simulink model "engine"  (R2019b)
settings: Solver=VariableStepAuto  StartTime=0.0  StopTime=9  MaxStep=1e-2  RelTol=1e-3
libraries: cstblocks x18, simulink x1
(part 1 of 2)
settings Model: PauseTimes=50  PacingRate=3  OrderedModelArguments=off  Creator=lenovo  LastModifiedBy=lenovo

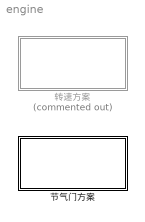
== system engine ==
  节气门方案 : Subsystem
  转速方案 : Subsystem  Commented=on

== system engine/节气门方案 ==
  note: 各个功率条件下，需要寻找功率随节气门开度变化斜率一致的转速
      | 详见转速-功率标定模块注释
  Gain : Gain  Gain=-1
  Gain1 : Gain  Gain=1e3
  Manual Switch1 : ManualSwitch
  Mux1 : Mux  Inputs=2
  Rate Limiter : RateLimiter  RisingSlewLimit=500  FallingSlewLimit=-500  SampleTimeMode=inherited
  Rate Limiter1 : RateLimiter  RisingSlewLimit=2000  FallingSlewLimit=-2000  SampleTimeMode=inherited
  Scope : Scope  NumInputPorts=4
  Sine Wave : Sin  Amplitude=10  Bias=20  Frequency=2*pi*0.01  SampleTime=0
  功率反馈补偿 : Subsystem
  功率设定 : Step  Time=3  Before=15  After=20  SampleTime=0
  功率闭环 : Subsystem  mask{Acc_p=1, Acc_n=1, Kp=3, Ki=0, Kd=0.01, D_Fc=2}
      mask prompts: Acc_p "最大正向加速度"; Acc_n "最大负向加速度"; Kp "PID-P"; Ki "PID-I"; Kd "PID-D"; D_Fc "PID-微分截止频率"
  发电机 : Subsystem
  总行程时间 : Constant  Value=3
  汽油机 : Subsystem
  电动油门 : Subsystem  mask{Deadband=1}
      mask prompts: Deadband "机械间隙（油门百分比）"
  转速-功率曲线 : Lookup_n-D  NumberOfTableDimensions=1  BreakpointsForDimension1=[0,4200,5600,6600,12500,14500,20000,26200,30500,33000]  BreakpointsForDimension2=[1:3]  Table=[800,800,860.1641,922.0328,1396.2121,1589.3308,2190.3409,2826.7045,3500,4000]  InternalRulePriority=Speed  RndMeth=Simplest  InputSameDT=on
  转速-功率标定 : Subsystem  Commented=on
  转速闭环 : Subsystem  mask{Trq_p=0, Trq_n=500, Kp=0.5, Ki=0.3, Kd=0.003, D_Fc=10}
      mask prompts: Trq_p "最大驱动扭矩"; Trq_n "最大发电扭矩"; Kp "PID-P"; Ki "PID-I"; Kd "PID-D"; D_Fc "PID-微分截止频率"
  wires:
  发电机/1(实际发电功率) -> Mux1/1, 转速-功率标定/1(发电功率)
  发电机/3(转速反馈) -> 功率反馈补偿/2(转速反馈), 转速闭环/1(转速反馈)
  发电机/2(电机实际扭矩) -> Gain/1
  汽油机/1(Speed) -> Scope/2, 发电机/1(转速)  "rpm"
  Gain/1 -> Scope/3, 汽油机/2(Load)  "负载"
  发电机/4(功率反馈) -> 功率反馈补偿/1(功率反馈)
  功率反馈补偿/1(补偿输出) -> 功率闭环/2(功率反馈)
  Gain1/1 -> Rate Limiter1/1
  Mux1/1 -> Scope/4  "功率"
  总行程时间/1 -> 电动油门/1(总行程时间)
  Rate Limiter1/1 -> 转速-功率曲线/1, 功率闭环/1(功率设定), Mux1/2
  功率闭环/1(节气门变化率输出) -> 电动油门/2(转速设定)  "油门信号"
  电动油门/1(节气门开度) -> Scope/1, 汽油机/1(Throttle)  "油门"
  转速闭环/1(扭矩输出) -> 发电机/2(扭矩设定)
  转速-功率曲线/1 -> Rate Limiter/1
  Rate Limiter/1 -> 转速闭环/2(转速设定)
  Sine Wave/1 -> Manual Switch1/1
  功率设定/1 -> Manual Switch1/2
  Manual Switch1/1 -> Gain1/1

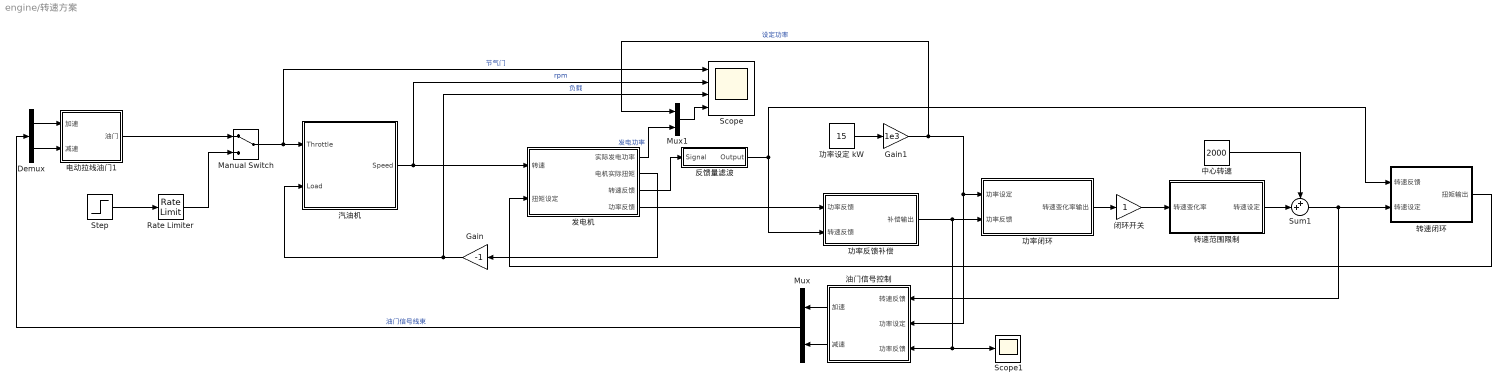
== system engine/转速方案 ==
  Demux : Demux  Outputs=2
  Gain : Gain  Gain=-1
  Gain1 : Gain  Gain=1e3
  Manual Switch : ManualSwitch
  Mux : Mux  Inputs=2
  Mux1 : Mux  Inputs=2
  Rate Limiter : RateLimiter  RisingSlewLimit=0.002  FallingSlewLimit=-0.002  SampleTimeMode=inherited
  Scope : Scope  NumInputPorts=4
  Scope1 : Scope
  Step : Step  Time=5  Before=0.2  After=0.4  SampleTime=0
  Sum1 : Sum  Inputs=++|
  中心转速 : Constant  Value=2000
  功率反馈补偿 : Subsystem
  功率设定 kW : Constant  Value=15
  功率闭环 : Subsystem  mask{Acc_p=500, Acc_n=500, Kp=0.4, Ki=0.2, Kd=0, D_Fc=20}
      mask prompts: Acc_p "最大正向加速度"; Acc_n "最大负向加速度"; Kp "PID-P"; Ki "PID-I"; Kd "PID-D"; D_Fc "PID-微分截止频率"
  反馈量滤波 : Subsystem  mask{Frq=20, Order=1}
      mask prompts: Frq "Frq_Set"; Order "Order_Set"
  发电机 : Subsystem
  汽油机 : Subsystem
  油门信号控制 : Subsystem
  电动拉线油门1 : Subsystem
  转速范围限制 : Subsystem  mask{Spe_Add=1000, Spe_Sub=1000}
      mask prompts: Spe_Add "最大转速增加量"; Spe_Sub "最大转速减少量"
  转速闭环 : Subsystem  mask{Trq_p=-10, Trq_n=500, Kp=0.8, Ki=0.7, Kd=0.005, D_Fc=20}
      mask prompts: Trq_p "最大驱动扭矩"; Trq_n "最大发电扭矩"; Kp "PID-P"; Ki "PID-I"; Kd "PID-D"; D_Fc "PID-微分截止频率"
  闭环开关 : Gain
  wires:
  Sum1/1 -> 油门信号控制/1(转速反馈), 转速闭环/2(转速设定)
  Step/1 -> Rate Limiter/1
  Mux1/1 -> Scope/4
  Gain1/1 -> Mux1/1, 功率闭环/1(功率设定), 油门信号控制/2(功率设定)  "设定功率"
  Rate Limiter/1 -> Manual Switch/2
  Manual Switch/1 -> Scope/1, 汽油机/1(Throttle)  "节气门"
  功率反馈补偿/1(补偿输出) -> 功率闭环/2(功率反馈), Scope1/1, 油门信号控制/3(功率反馈)
  油门信号控制/2(减速) -> Mux/2
  Mux/1 -> Demux/1  "油门信号线束"
  油门信号控制/1(加速) -> Mux/1
  发电机/4(功率反馈) -> 功率反馈补偿/1(功率反馈)
  闭环开关/1 -> 转速范围限制/1(转速变化率)
  Gain/1 -> 汽油机/2(Load), Scope/3  "负载"
  汽油机/1(Speed) -> Scope/2, 发电机/1(转速)  "rpm"
  发电机/2(电机实际扭矩) -> Gain/1
  发电机/3(转速反馈) -> 反馈量滤波/1(Signal)
  Demux/2 -> 电动拉线油门1/2(减速)
  转速闭环/1(扭矩输出) -> 发电机/2(扭矩设定)
  Demux/1 -> 电动拉线油门1/1(加速)
  反馈量滤波/1(Output) -> 转速闭环/1(转速反馈), 功率反馈补偿/2(转速反馈)
  功率闭环/1(转速变化率输出) -> 闭环开关/1
  中心转速/1 -> Sum1/1
  转速范围限制/1(转速设定) -> Sum1/2
  功率设定 kW/1 -> Gain1/1
  电动拉线油门1/1(油门) -> Manual Switch/1
  发电机/1(实际发电功率) -> Mux1/2  "发电功率"

== system engine/节气门方案/功率反馈补偿 ==
  note: 通过计算，将控制发动机加减速消耗的功率从功率反馈量中剔除
  note: 反馈系数：
      | 通过调整反馈系数，完全抵消转速变化时的动能变化对功率反馈的影响
      | 节气门不变，转速提高时用于反馈的功率应单调增大
      | 由于加减速时发动机工况有差异，此处反馈系数仅根据发动机转动惯量计算反馈补偿量不够准确，
      | 需要调参使得反馈效果最好。
  功率反馈 : Inport
  转速反馈 : Inport  Port=2
  Derivative : Derivative  CoefficientInTFapproximation=0.1
  Gain1 : Gain  Gain=pi/30
  Mux : Mux  Inputs=2
  Scope2 : Scope  NumInputPorts=3
  Sum : Sum  Inputs=++|
  功率反馈滤波 : Subsystem  mask{Frq=20, Order=1}
      mask prompts: Frq "Frq_Set"; Order "Order_Set"
  功率反馈补偿后滤波 : Subsystem  mask{Frq=10, Order=5}
      mask prompts: Frq "Frq_Set"; Order "Order_Set"
  反馈系数 : Gain  Gain=0.8
  转动动能 : Fcn  Expr=0.5*u(2)*u(1)*u(1)
  转动惯量 : Constant  Value=0.25
  补偿输出 : Outport
  wires:
  功率反馈/1 -> 功率反馈滤波/1(Signal)
  转动惯量/1 -> Mux/2
  Derivative/1 -> 反馈系数/1
  转速反馈/1 -> Gain1/1
  功率反馈滤波/1(Output) -> Scope2/1, Sum/1
  Mux/1 -> 转动动能/1
  转动动能/1 -> Derivative/1
  反馈系数/1 -> Sum/2, Scope2/2
  Sum/1 -> 功率反馈补偿后滤波/1(Signal)
  Gain1/1 -> Mux/1
  功率反馈补偿后滤波/1(Output) -> Scope2/3, 补偿输出/1

== system engine/节气门方案/功率闭环 ==
  功率设定 : Inport
  功率反馈 : Inport  Port=2
  Kd : Gain  Gain=Kd
  Ki : Gain  Gain=Ki
  Kp : Gain  Gain=Kp
  Product : Product  Inputs=**
  Saturation : Saturate  UpperLimit=Acc_p  LowerLimit=-Acc_n
  Sum : Sum  Inputs=|+-
  Sum1 : Sum  Inputs=+++
  Zero-Order Hold : ZeroOrderHold  SampleTime=0.01
  微分 : Subsystem  mask{fc_Set=D_Fc}
      mask prompts: fc_Set "截止频率（fc）"
  数量级调整 : Gain  Gain=1e-4
  积分:限制正扭矩 : Integrator  LimitOutput=on  UpperSaturationLimit=Acc_p  LowerSaturationLimit=-Acc_n
  积分控制 : Subsystem  mask{dPWR=10000}
      mask prompts: dPWR "停止积分的功率斜率 W/s"
  节气门变化率输出 : Outport
  wires:
  Kd/1 -> 微分/1(Err)
  微分/1(dErr) -> Sum1/3
  积分控制/1(开启积分) -> Product/2
  Sum/1 -> 数量级调整/1  "Error"
  Ki/1 -> Product/1
  Product/1 -> 积分:限制正扭矩/1
  Saturation/1 -> 节气门变化率输出/1
  积分:限制正扭矩/1 -> Sum1/2
  Kp/1 -> Sum1/1
  功率设定/1 -> Sum/1
  功率反馈/1 -> Sum/2
  Sum1/1 -> Zero-Order Hold/1, 积分控制/2(Output)
  数量级调整/1 -> 积分控制/1(Error), Kd/1, Ki/1, Kp/1
  Zero-Order Hold/1 -> Saturation/1

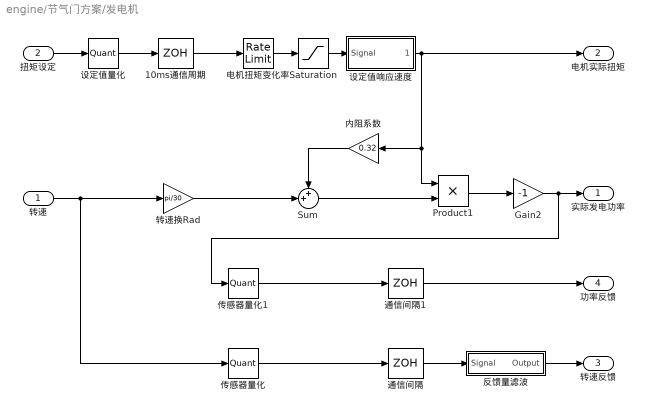
== system engine/节气门方案/发电机 ==
  转速 : Inport
  扭矩设定 : Inport  Port=2
  10ms通信周期 : ZeroOrderHold  SampleTime=0.01
  Gain2 : Gain  Gain=-1
  Product1 : Product
  Saturation : Saturate  UpperLimit=500  LowerLimit=-500
  Sum : Sum  Inputs=++|
  传感器量化 : Quantizer
  传感器量化1 : Quantizer
  内阻系数 : Gain  Gain=0.32
  反馈量滤波 : Subsystem  mask{Frq=25, Order=1}
      mask prompts: Frq "Frq_Set"; Order "Order_Set"
  电机扭矩变化率 : RateLimiter  RisingSlewLimit=5000  FallingSlewLimit=-5000  SampleTimeMode=inherited
  设定值响应速度 : Subsystem  mask{Frq=100, Order=1}
      mask prompts: Frq "Frq_Set"; Order "Order_Set"
  设定值量化 : Quantizer  QuantizationInterval=0.1
  转速换Rad : Gain  Gain=pi/30
  通信间隔 : ZeroOrderHold  SampleTime=0.01
  通信间隔1 : ZeroOrderHold  SampleTime=0.01
  实际发电功率 : Outport
  电机实际扭矩 : Outport  Port=2
  转速反馈 : Outport  Port=3
  功率反馈 : Outport  Port=4
  wires:
  通信间隔1/1 -> 功率反馈/1
  传感器量化1/1 -> 通信间隔1/1
  设定值量化/1 -> 10ms通信周期/1
  扭矩设定/1 -> 设定值量化/1
  传感器量化/1 -> 通信间隔/1
  Saturation/1 -> 设定值响应速度/1(Signal)
  10ms通信周期/1 -> 电机扭矩变化率/1
  Gain2/1 -> 传感器量化1/1, 实际发电功率/1
  电机扭矩变化率/1 -> Saturation/1
  Sum/1 -> Product1/2
  内阻系数/1 -> Sum/1
  转速换Rad/1 -> Sum/2
  转速/1 -> 转速换Rad/1, 传感器量化/1
  Product1/1 -> Gain2/1
  设定值响应速度/1(Output) -> 电机实际扭矩/1, 内阻系数/1, Product1/1
  通信间隔/1 -> 反馈量滤波/1(Signal)
  反馈量滤波/1(Output) -> 转速反馈/1

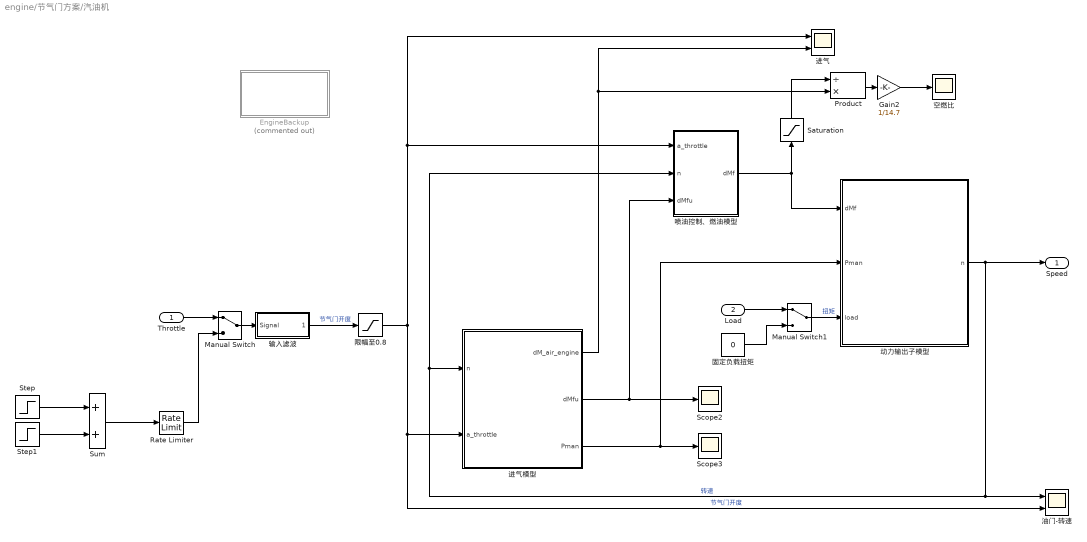
== system engine/节气门方案/汽油机 ==
  Throttle : Inport
  Load : Inport  Port=2
  EngineBackup : Subsystem  Commented=on
  Gain2 : Gain  Gain=1/14.7  SaturateOnIntegerOverflow=on  OutDataTypeStr=Inherit: Same as input  ParamDataTypeStr=Inherit: Same as input
  Manual Switch : ManualSwitch
  Manual Switch1 : ManualSwitch
  Product : Product  Inputs=/*  SaturateOnIntegerOverflow=on  OutDataTypeStr=Inherit: Same as first input
  Rate Limiter : RateLimiter  RisingSlewLimit=0.2  FallingSlewLimit=-0.2  SampleTimeMode=inherited
  Saturation : Saturate  UpperLimit=1e6  LowerLimit=1e-6
  Scope2 : Scope
  Scope3 : Scope
  Step : Step  Time=30  After=-0.1  SampleTime=0
  Step1 : Step  Time=5  Before=0.1  After=0.2  SampleTime=0
  Sum : Sum
  动力输出子模型 : Subsystem  mask{Ie=0.25}
      mask prompts: Ie "转动惯量（Ie）"
  喷油控制、燃油模型 : Subsystem
  固定负载扭矩 : Constant  Value=0
  油门-转速 : Scope  NumInputPorts=2
  空燃比 : Scope
  输入滤波 : Subsystem  mask{Frq=20, Order=1}
      mask prompts: Frq "Frq_Set"; Order "Order_Set"
  进气 : Scope  NumInputPorts=2
  进气模型 : Subsystem
  限幅至0.8 : Saturate  UpperLimit=0.8  LowerLimit=0
  Speed : Outport
  wires:
  限幅至0.8/1 -> 喷油控制、燃油模型/1(a_throttle), 进气/1, 油门-转速/2, 进气模型/2(a_throttle)  "节气门开度"
  Manual Switch/1 -> 输入滤波/1(Signal)
  Step1/1 -> Sum/2
  Step/1 -> Sum/1
  Manual Switch1/1 -> 动力输出子模型/3(load)  "扭矩"
  Load/1 -> Manual Switch1/1
  Rate Limiter/1 -> Manual Switch/2
  Throttle/1 -> Manual Switch/1
  输入滤波/1(Output) -> 限幅至0.8/1  "节气门开度"
  Saturation/1 -> Product/1
  进气模型/3(Pman) -> Scope3/1, 动力输出子模型/2(Pman)
  Gain2/1 -> 空燃比/1
  固定负载扭矩/1 -> Manual Switch1/2
  动力输出子模型/1(n) -> 油门-转速/1, 喷油控制、燃油模型/2(n), 进气模型/1(n), Speed/1  "转速"
  Sum/1 -> Rate Limiter/1
  喷油控制、燃油模型/1(dMf) -> 动力输出子模型/1(dMf), Saturation/1
  Product/1 -> Gain2/1
  进气模型/2(dMfu) -> 喷油控制、燃油模型/3(dMfu), Scope2/1
  进气模型/1("dM_air_engine ") -> Product/2, 进气/2

== system engine/节气门方案/电动油门 ==
  总行程时间 : Inport
  转速设定 : Inport  Port=2
  Integrator : Integrator  LimitOutput=on  UpperSaturationLimit=1  LowerSaturationLimit=0
  Integrator1 : Integrator  LimitOutput=on  UpperSaturationLimit=1  LowerSaturationLimit=-1
  PID Controller : simulink/Continuous/PID Controller  Controller=PID  Form=Parallel  TimeDomain=Continuous-time  SampleTime=-1  IntegratorMethod=Forward Euler  FilterMethod=Forward Euler  ControllerParametersSource=internal  P=10  I=0  D=0  UseFilter=on  N=100  TunerSelectOption=Transfer Function Based (PID Tuner App)  InitialConditionSource=internal  InitialConditionForIntegrator=0  InitialConditionForFilter=0  DifferentiatorICPrevScaledInput=0  ExternalReset=none  TrackingMode=off  Kt=1  LimitOutput=on  UpperSaturationLimit=5  LowerSaturationLimit=-5  LinearizeAsGain=on  AntiWindupMode=none  Kb=1  POutMin=[]  POutMax=[]  IOutMin=[]  IOutMax=[]  DOutMin=[]  DOutMax=[]  NOutMin=[]  NOutMax=[]  SumOutMin=[]  SumOutMax=[]  SaturationOutMin=[]  SaturationOutMax=[]  PParamMin=[]  PParamMax=[]  IParamMin=[]  IParamMax=[]  DParamMin=[]  DParamMax=[]  NParamMin=[]  NParamMax=[]  KbParamMin=[]  KbParamMax=[]  KtParamMin=[]  KtParamMax=[]  KbOutMin=[]  KbOutMax=[]  KtOutMin=[]  KtOutMax=[]  IntegratorOutMin=[]  IntegratorOutMax=[]  FilterOutMin=[]  FilterOutMax=[]  SumI1OutMin=[]  SumI1OutMax=[]  SumI2OutMin=[]  SumI2OutMax=[]  SumI3OutMin=[]  SumI3OutMax=[]  SumI4OutMin=[]  SumI4OutMax=[]  SumDOutMin=[]  SumDOutMax=[]  DifferentiatorOutMin=[]  DifferentiatorOutMax=[]  FilterDiffOutCoefMin=[]  FilterDiffOutCoefMax=[]  ReciprocalOutMin=[]  ReciprocalOutMax=[]  SumDenOutMin=[]  SumDenOutMax=[]  SumNumOutMin=[]  SumNumOutMax=[]  DivideOutMin=[]  DivideOutMax=[]  IntegratorContinuousStateAttributes=''  IntegratorStateMustResolveToSignalObject=off  IntegratorRTWStateStorageClass=Auto  FilterContinuousStateAttributes=''  FilterStateMustResolveToSignalObject=off  FilterRTWStateStorageClass=Auto  ParallelPVariant=InternalParameters  IdealPVariant=Disabled  IVariant=InternalParameters  DVariant=InternalParameters  IntegratorVariant=Continuous  SatVariant=Enabled  AWVariant=Passthrough  PCopyVariant=Disabled  TRVariant=Disabled  FdbkBlocksVariant=Forward  IdealPFdbkVariant=Disabled  SatFdbkVariant=Disabled  DerivativeFilterVariant=ContFilter  NVariant=InternalParameters  NCopyVariant=Disabled  FilterICVariant=InternalICsFilter  IntegratorICVariant=InternalICs  ExternalResetVariant=Disabled  TRSumVariant=Passthrough  SumFdbkVariant=Disabled  SumVariant=Sum_PID
  Product : Product  Inputs=*/
  Saturation : Saturate  UpperLimit=1  LowerLimit=-1
  Sum : Sum  Inputs=|++
  Sum2 : Sum  Inputs=|+-
  减轻仿真负担 : Memory
  最小油门 : Constant  Value=0
  油门行程 : Gain  Gain=0.8
  滞后 : Subsystem  mask{Frq=500, Order=3}
      mask prompts: Frq "Frq_Set"; Order "Order_Set"
  通信量化 : Quantizer  QuantizationInterval=0.001
  间隙 : Backlash  BacklashWidth=Deadband/100
  节气门开度 : Outport
  wires:
  Product/1 -> Integrator/1
  Integrator1/1 -> Sum2/2, Product/1  "实际转速"
  Integrator/1 -> 油门行程/1
  Sum2/1 -> PID Controller/1
  油门行程/1 -> Sum/1
  滞后/1(Output) -> Sum2/1
  PID Controller/1 -> Integrator1/1
  Sum/1 -> 间隙/1
  最小油门/1 -> Sum/2
  Saturation/1 -> 滞后/1(Signal)
  总行程时间/1 -> Product/2
  转速设定/1 -> 通信量化/1
  通信量化/1 -> Saturation/1
  间隙/1 -> 减轻仿真负担/1
  减轻仿真负担/1 -> 节气门开度/1

== system engine/节气门方案/转速-功率标定 ==
  note: 原理：
      | 这里的功率变化率X对应功率闭环的执行器的灵敏度，在不同转速不同功率的情况下，选取了相同的X，则不同转速时，功率闭环的执行器具有较好的一致性。
      | X的值选取在峰值出现后一段时间，因为峰值对应着发动机机械效率的激增，峰值时刻发动机机械效率还没有增大到比较大的值，而峰值后一段时间，
      | 对应着发动机机械效率已经上升到较高水平，但随节气门开度变化仍有一定上升空间，此时最能兼顾控制需求与效率需求。
  note: 标定方法：
      | 直接指定转速闭环设定值，每间隔一定转速标定一轮
      | 每轮标定中，需要将节气门开度随时间匀速缓慢增大，
      | 观察发电功率变化率随节气门开度的变化情况，变化曲线中会包含一个峰值，
      | 这里选取峰值时刻之后一段时间的某一时刻，此时变化曲线已经比较平缓，此时刻的功率变化率记为X
      | 每轮标定中选取的X需相近。
      | 选定使得功率变化率为X的时刻后，查看该时刻的功率，该功率即与本轮标定的转速相对应。
  发电功率 : Inport
  Scope2 : Scope
  Scope3 : Scope
  Subsystem1 : Subsystem
  wires:
  发电功率/1 -> Scope2/1, Subsystem1/1(发电功率)
  Subsystem1/1(控制斜率) -> Scope3/1

== system engine/节气门方案/转速闭环 ==
  转速反馈 : Inport
  转速设定 : Inport  Port=2
  Kd : Gain  Gain=Kd
  Ki : Gain  Gain=Ki
  Kp : Gain  Gain=Kp
  Product : Product  Inputs=**
  Saturation : Saturate  UpperLimit=Trq_p  LowerLimit=-Trq_n
  Sum : Sum  Inputs=|+-
  Sum1 : Sum  Inputs=+++
  Zero-Order Hold : ZeroOrderHold  SampleTime=0.01
  微分 : Subsystem  mask{fc_Set=D_Fc}
      mask prompts: fc_Set "截止频率（fc）"
  积分:限制正扭矩 : Integrator  InitialCondition=Trq_p  LimitOutput=on  UpperSaturationLimit=Trq_p  LowerSaturationLimit=-Trq_n
  积分控制 : Subsystem  mask{dRPM=1000}
      mask prompts: dRPM "停止积分的转速斜率 rpm/s"
  扭矩输出 : Outport
  wires:
  Kd/1 -> 微分/1(Err)
  微分/1(dErr) -> Sum1/3
  积分控制/1(开启积分) -> Product/2
  Sum/1 -> 积分控制/1(Error), Kd/1, Ki/1, Kp/1  "Error"
  Ki/1 -> Product/1
  Product/1 -> 积分:限制正扭矩/1
  Saturation/1 -> 扭矩输出/1
  积分:限制正扭矩/1 -> Sum1/2
  Kp/1 -> Sum1/1
  转速设定/1 -> Sum/1
  转速反馈/1 -> Sum/2
  Sum1/1 -> 积分控制/2(Output), Zero-Order Hold/1
  Zero-Order Hold/1 -> Saturation/1

== system engine/转速方案/功率反馈补偿 ==
  note: 反馈系数：
      | 通过调整反馈系数，完全抵消转速变化时的动能变化对功率反馈的影响
      | 节气门不变，转速提高时用于反馈的功率应单调增大
      | 由于加减速时发动机工况有差异，此处反馈系数仅根据发动机转动惯量计算反馈补偿量不够准确，
      | 需要调参使得反馈效果最好。
  note: 通过计算，将控制发动机加减速消耗的功率从功率反馈量中剔除
  功率反馈 : Inport
  转速反馈 : Inport  Port=2
  Derivative : Derivative  CoefficientInTFapproximation=0.1
  Gain1 : Gain  Gain=pi/30
  Mux : Mux  Inputs=2
  Scope2 : Scope  NumInputPorts=3
  Sum : Sum  Inputs=++|
  功率反馈滤波 : Subsystem  mask{Frq=20, Order=1}
      mask prompts: Frq "Frq_Set"; Order "Order_Set"
  功率反馈补偿后滤波 : Subsystem  mask{Frq=10, Order=5}
      mask prompts: Frq "Frq_Set"; Order "Order_Set"
  反馈系数 : Gain  Gain=0.7
  转动动能 : Fcn  Expr=0.5*u(2)*u(1)*u(1)
  转动惯量 : Constant  Value=0.25
  补偿输出 : Outport
  wires:
  功率反馈补偿后滤波/1(Output) -> 补偿输出/1, Scope2/3
  Gain1/1 -> Mux/1
  Sum/1 -> 功率反馈补偿后滤波/1(Signal)
  反馈系数/1 -> Scope2/2, Sum/2
  转动动能/1 -> Derivative/1
  Mux/1 -> 转动动能/1
  功率反馈滤波/1(Output) -> Sum/1, Scope2/1
  转速反馈/1 -> Gain1/1
  Derivative/1 -> 反馈系数/1
  转动惯量/1 -> Mux/2
  功率反馈/1 -> 功率反馈滤波/1(Signal)

== system engine/转速方案/功率闭环 ==
  功率设定 : Inport
  功率反馈 : Inport  Port=2
  Kd : Gain  Gain=Kd
  Ki : Gain  Gain=Ki
  Kp : Gain  Gain=Kp
  Product : Product  Inputs=**
  Saturation : Saturate  UpperLimit=Acc_p  LowerLimit=-Acc_n
  Sum : Sum  Inputs=|+-
  Sum1 : Sum  Inputs=+++
  微分 : Subsystem  mask{fc_Set=D_Fc}
      mask prompts: fc_Set "截止频率（fc）"
  积分:限制正扭矩 : Integrator  LimitOutput=on  UpperSaturationLimit=Acc_p  LowerSaturationLimit=-Acc_n
  积分控制 : Subsystem  mask{dPWR=10000}
      mask prompts: dPWR "停止积分的功率斜率 W/s"
  转速变化率输出 : Outport
  wires:
  Kd/1 -> 微分/1(Err)
  微分/1(dErr) -> Sum1/3
  积分控制/1(开启积分) -> Product/2
  Sum/1 -> 积分控制/1(Error), Kd/1, Ki/1, Kp/1  "Error"
  Ki/1 -> Product/1
  Product/1 -> 积分:限制正扭矩/1
  Saturation/1 -> 转速变化率输出/1
  积分:限制正扭矩/1 -> Sum1/2
  Kp/1 -> Sum1/1
  功率设定/1 -> Sum/1
  功率反馈/1 -> Sum/2
  Sum1/1 -> Saturation/1, 积分控制/2(Output)

== system engine/转速方案/反馈量滤波 ==
  Signal : Inport
  Constant2 : Constant  Value=Frq
  Gain : Gain  Gain=2*pi
  d_Smp_LPF6 : cstblocks/Linear Parameter Varying/Varying Lowpass Filter  N=Order
      settings: SourceProductName=Control System Toolbox
  Output : Outport
  wires:
  d_Smp_LPF6/1 -> Output/1  "Is"
  Constant2/1 -> Gain/1
  Signal/1 -> d_Smp_LPF6/1
  Gain/1 -> d_Smp_LPF6/2

== system engine/转速方案/发电机 ==
  转速 : Inport
  扭矩设定 : Inport  Port=2
  10ms通信周期 : ZeroOrderHold  SampleTime=0.01
  Gain2 : Gain  Gain=-1
  Product1 : Product
  Saturation : Saturate  UpperLimit=500  LowerLimit=-500
  Sum : Sum  Inputs=++|
  传感器量化 : Quantizer
  传感器量化1 : Quantizer
  内阻系数 : Gain  Gain=0.32
  电机扭矩变化率 : RateLimiter  RisingSlewLimit=5000  FallingSlewLimit=-5000  SampleTimeMode=inherited
  设定值响应速度 : Subsystem  mask{Frq=100, Order=1}
      mask prompts: Frq "Frq_Set"; Order "Order_Set"
  设定值量化 : Quantizer  QuantizationInterval=0.1
  转速换Rad : Gain  Gain=pi/30
  通信间隔 : ZeroOrderHold  SampleTime=0.01
  通信间隔1 : ZeroOrderHold  SampleTime=0.01
  实际发电功率 : Outport
  电机实际扭矩 : Outport  Port=2
  转速反馈 : Outport  Port=3
  功率反馈 : Outport  Port=4
  wires:
  设定值响应速度/1(Output) -> Product1/1, 内阻系数/1, 电机实际扭矩/1
  Product1/1 -> Gain2/1
  转速/1 -> 传感器量化/1, 转速换Rad/1
  转速换Rad/1 -> Sum/2
  内阻系数/1 -> Sum/1
  Sum/1 -> Product1/2
  电机扭矩变化率/1 -> Saturation/1
  Gain2/1 -> 实际发电功率/1, 传感器量化1/1
  10ms通信周期/1 -> 电机扭矩变化率/1
  Saturation/1 -> 设定值响应速度/1(Signal)
  传感器量化/1 -> 通信间隔/1
  通信间隔/1 -> 转速反馈/1
  扭矩设定/1 -> 设定值量化/1
  设定值量化/1 -> 10ms通信周期/1
  传感器量化1/1 -> 通信间隔1/1
  通信间隔1/1 -> 功率反馈/1

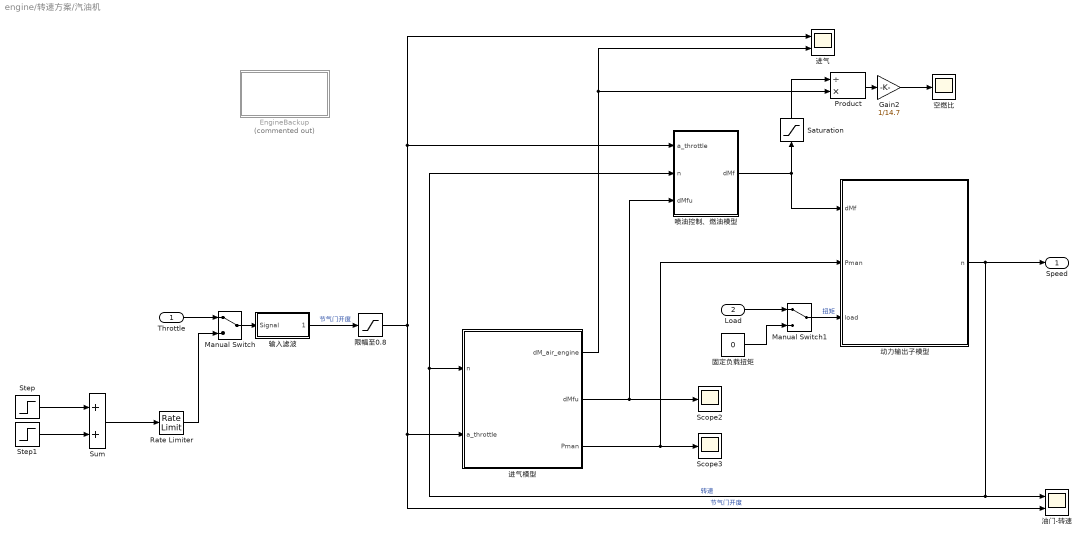
== system engine/转速方案/汽油机 ==
  Throttle : Inport
  Load : Inport  Port=2
  EngineBackup : Subsystem  Commented=on
  Gain2 : Gain  Gain=1/14.7  SaturateOnIntegerOverflow=on  OutDataTypeStr=Inherit: Same as input  ParamDataTypeStr=Inherit: Same as input
  Manual Switch : ManualSwitch
  Manual Switch1 : ManualSwitch
  Product : Product  Inputs=/*  SaturateOnIntegerOverflow=on  OutDataTypeStr=Inherit: Same as first input
  Rate Limiter : RateLimiter  RisingSlewLimit=0.2  FallingSlewLimit=-0.2  SampleTimeMode=inherited
  Saturation : Saturate  UpperLimit=1e6  LowerLimit=1e-6
  Scope2 : Scope
  Scope3 : Scope
  Step : Step  Time=30  After=-0.1  SampleTime=0
  Step1 : Step  Time=5  Before=0.1  After=0.2  SampleTime=0
  Sum : Sum
  动力输出子模型 : Subsystem  mask{Ie=0.25}
      mask prompts: Ie "转动惯量（Ie）"
  喷油控制、燃油模型 : Subsystem
  固定负载扭矩 : Constant  Value=0
  油门-转速 : Scope  NumInputPorts=2
  空燃比 : Scope
  输入滤波 : Subsystem  mask{Frq=20, Order=1}
      mask prompts: Frq "Frq_Set"; Order "Order_Set"
  进气 : Scope  NumInputPorts=2
  进气模型 : Subsystem
  限幅至0.8 : Saturate  UpperLimit=0.8  LowerLimit=0
  Speed : Outport
  wires:
  进气模型/1("dM_air_engine ") -> 进气/2, Product/2
  进气模型/2(dMfu) -> Scope2/1, 喷油控制、燃油模型/3(dMfu)
  Product/1 -> Gain2/1
  喷油控制、燃油模型/1(dMf) -> Saturation/1, 动力输出子模型/1(dMf)
  Sum/1 -> Rate Limiter/1
  动力输出子模型/1(n) -> Speed/1, 进气模型/1(n), 喷油控制、燃油模型/2(n), 油门-转速/1  "转速"
  固定负载扭矩/1 -> Manual Switch1/2
  Gain2/1 -> 空燃比/1
  进气模型/3(Pman) -> 动力输出子模型/2(Pman), Scope3/1
  Saturation/1 -> Product/1
  输入滤波/1(Output) -> 限幅至0.8/1  "节气门开度"
  Throttle/1 -> Manual Switch/1
  Rate Limiter/1 -> Manual Switch/2
  Load/1 -> Manual Switch1/1
  Manual Switch1/1 -> 动力输出子模型/3(load)  "扭矩"
  Step/1 -> Sum/1
  Step1/1 -> Sum/2
  Manual Switch/1 -> 输入滤波/1(Signal)
  限幅至0.8/1 -> 进气模型/2(a_throttle), 油门-转速/2, 进气/1, 喷油控制、燃油模型/1(a_throttle)  "节气门开度"

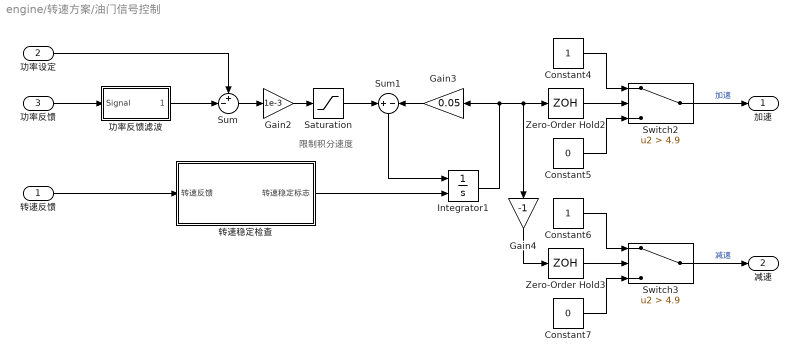
== system engine/转速方案/油门信号控制 ==
  note: 限制积分速度
  转速反馈 : Inport
  功率设定 : Inport  Port=2
  功率反馈 : Inport  Port=3
  Constant4 : Constant
  Constant5 : Constant  Value=0
  Constant6 : Constant
  Constant7 : Constant  Value=0
  Gain2 : Gain  Gain=1e-3
  Gain3 : Gain  Gain=0.05
  Gain4 : Gain  Gain=-1
  Integrator1 : Integrator  ExternalReset=level hold  LimitOutput=on  UpperSaturationLimit=5  LowerSaturationLimit=-5
  Saturation : Saturate  UpperLimit=5  LowerLimit=-5
  Sum : Sum  Inputs=+-|
  Sum1 : Sum  Inputs=+-
  Switch2 : Switch  Criteria=u2 > Threshold  Threshold=4.9
  Switch3 : Switch  Criteria=u2 > Threshold  Threshold=4.9
  Zero-Order Hold2 : ZeroOrderHold  SampleTime=0.01
  Zero-Order Hold3 : ZeroOrderHold  SampleTime=0.01
  功率反馈滤波 : Subsystem  mask{Frq=5, Order=5}
      mask prompts: Frq "Frq_Set"; Order "Order_Set"
  转速稳定检查 : Subsystem
  加速 : Outport
  减速 : Outport  Port=2
  wires:
  Gain4/1 -> Zero-Order Hold3/1
  Switch3/1 -> 减速/1  "减速"
  Sum/1 -> Gain2/1
  Constant6/1 -> Switch3/1
  功率反馈滤波/1(Output) -> Sum/2
  Constant7/1 -> Switch3/3
  Zero-Order Hold2/1 -> Switch2/2
  Integrator1/1 -> Zero-Order Hold2/1, Gain4/1, Gain3/1
  Zero-Order Hold3/1 -> Switch3/2
  Constant4/1 -> Switch2/1
  Switch2/1 -> 加速/1  "加速"
  Constant5/1 -> Switch2/3
  功率反馈/1 -> 功率反馈滤波/1(Signal)
  Gain2/1 -> Saturation/1
  功率设定/1 -> Sum/1
  转速反馈/1 -> 转速稳定检查/1(转速反馈)
  转速稳定检查/1(转速稳定标志) -> Integrator1/2
  Sum1/1 -> Integrator1/1
  Gain3/1 -> Sum1/2
  Saturation/1 -> Sum1/1

== system engine/转速方案/电动拉线油门1 ==
  加速 : Inport
  减速 : Inport  Port=2
  Constant3 : Constant
  Constant4 : Constant  Value=0
  Constant5 : Constant
  Constant6 : Constant  Value=0
  Product : Product  Inputs=*/
  Sum : Sum  Inputs=+-
  Sum1 : Sum  Inputs=|++
  Switch : Switch  Criteria=u2 > Threshold
  Switch1 : Switch  Criteria=u2 > Threshold
  最小油门 : Constant  Value=0.15
  油门可调范围 : Gain  Gain=0.2
  油门拉线位置 : Integrator  LimitOutput=on  UpperSaturationLimit=1  LowerSaturationLimit=0
  油门拉线完整行程耗时 : Constant  Value=10
  间隙 : Backlash  BacklashWidth=0.01
  驱动电机加速度限制1 : RateLimiter  RisingSlewLimit=5  FallingSlewLimit=-5  SampleTimeMode=inherited
  驱动电机加速度限制2 : RateLimiter  RisingSlewLimit=5  FallingSlewLimit=-5  SampleTimeMode=inherited
  油门 : Outport
  wires:
  油门可调范围/1 -> Sum1/1
  油门拉线完整行程耗时/1 -> Product/2
  Product/1 -> 油门拉线位置/1
  间隙/1 -> 油门可调范围/1
  驱动电机加速度限制2/1 -> Sum/2
  驱动电机加速度限制1/1 -> Sum/1
  Switch1/1 -> 驱动电机加速度限制2/1
  Constant4/1 -> Switch/3
  Constant6/1 -> Switch1/3
  Constant3/1 -> Switch/1
  Switch/1 -> 驱动电机加速度限制1/1
  油门拉线位置/1 -> 间隙/1
  加速/1 -> Switch/2
  Sum/1 -> Product/1
  Constant5/1 -> Switch1/1
  减速/1 -> Switch1/2
  Sum1/1 -> 油门/1
  最小油门/1 -> Sum1/2

== system engine/转速方案/转速范围限制 ==
  转速变化率 : Inport
  Integrator : Integrator  LimitOutput=on  UpperSaturationLimit=Spe_Add  LowerSaturationLimit=-Spe_Sub
  转速设定 : Outport
  wires:
  转速变化率/1 -> Integrator/1
  Integrator/1 -> 转速设定/1

== system engine/转速方案/转速闭环 ==
  转速反馈 : Inport
  转速设定 : Inport  Port=2
  Kd : Gain  Gain=Kd
  Ki : Gain  Gain=Ki
  Kp : Gain  Gain=Kp
  Product : Product  Inputs=**
  Saturation : Saturate  UpperLimit=Trq_p  LowerLimit=-Trq_n
  Sum : Sum  Inputs=|+-
  Sum1 : Sum  Inputs=+++
  微分 : Subsystem  mask{fc_Set=D_Fc}
      mask prompts: fc_Set "截止频率（fc）"
  积分:限制正扭矩 : Integrator  InitialCondition=Trq_p  LimitOutput=on  UpperSaturationLimit=Trq_p  LowerSaturationLimit=-Trq_n
  积分控制 : Subsystem  mask{dRPM=1000}
      mask prompts: dRPM "停止积分的转速斜率 rpm/s"
  扭矩输出 : Outport
  wires:
  Sum1/1 -> Saturation/1, 积分控制/2(Output)
  转速反馈/1 -> Sum/2
  转速设定/1 -> Sum/1
  Kp/1 -> Sum1/1
  积分:限制正扭矩/1 -> Sum1/2
  Saturation/1 -> 扭矩输出/1
  Product/1 -> 积分:限制正扭矩/1
  Ki/1 -> Product/1
  Sum/1 -> Kp/1, Ki/1, Kd/1, 积分控制/1(Error)  "Error"
  积分控制/1(开启积分) -> Product/2
  微分/1(dErr) -> Sum1/3
  Kd/1 -> 微分/1(Err)

== system engine/节气门方案/功率反馈补偿/功率反馈滤波 ==
  Signal : Inport
  Constant2 : Constant  Value=Frq
  Gain : Gain  Gain=2*pi
  d_Smp_LPF6 : cstblocks/Linear Parameter Varying/Varying Lowpass Filter  N=Order
      settings: SourceProductName=Control System Toolbox
  Output : Outport
  wires:
  Gain/1 -> d_Smp_LPF6/2
  Signal/1 -> d_Smp_LPF6/1
  Constant2/1 -> Gain/1
  d_Smp_LPF6/1 -> Output/1  "Is"

== system engine/节气门方案/功率反馈补偿/功率反馈补偿后滤波 ==
  Signal : Inport
  Constant2 : Constant  Value=Frq
  Gain : Gain  Gain=2*pi
  d_Smp_LPF6 : cstblocks/Linear Parameter Varying/Varying Lowpass Filter  N=Order
      settings: SourceProductName=Control System Toolbox
  Output : Outport
  wires:
  d_Smp_LPF6/1 -> Output/1  "Is"
  Constant2/1 -> Gain/1
  Signal/1 -> d_Smp_LPF6/1
  Gain/1 -> d_Smp_LPF6/2

== system engine/节气门方案/功率闭环/微分 ==
  Err : Inport
  Derivative : Derivative  CoefficientInTFapproximation=0.1
  微分滤波1 : Subsystem  mask{Frq=fc_Set, Order=1}
      mask prompts: Frq "Frq_Set"; Order "Order_Set"
  dErr : Outport
  wires:
  Derivative/1 -> dErr/1
  微分滤波1/1(Output) -> Derivative/1
  Err/1 -> 微分滤波1/1(Signal)

== system engine/节气门方案/功率闭环/积分控制 ==
  note: 功率快速增大时积分不增大
      | 功率快速减小时积分不减小
  Error : Inport
  Output : Inport  Port=2
  Derivative : Derivative  CoefficientInTFapproximation=0.1
  Memory : Memory
  Memory1 : Memory
  Product1 : Product  Inputs=3
  Scope : Scope  NumInputPorts=3
  Subsystem : Subsystem
  Zero-Order Hold : ZeroOrderHold  SampleTime=0.01
  Zero-Order Hold1 : ZeroOrderHold  SampleTime=0.01
  Zero-Order Hold2 : ZeroOrderHold  SampleTime=0.01
  输出达到正限幅时积分不再增大 : Subsystem
  输出达到负限幅时积分不再减小 : Subsystem
  开启积分 : Outport
  wires:
  Subsystem/1(启动积分) -> Product1/1, Scope/1  "斜率限制"
  Zero-Order Hold1/1 -> Subsystem/1(dErr)
  Zero-Order Hold2/1 -> Memory1/1
  Derivative/1 -> Zero-Order Hold1/1
  Zero-Order Hold/1 -> Memory/1
  输出达到正限幅时积分不再增大/1(启动积分) -> Product1/2, Scope/2  "正限幅限制"
  输出达到负限幅时积分不再减小/1(启动积分) -> Product1/3, Scope/3  "负限幅限制"
  Output/1 -> Zero-Order Hold2/1
  Product1/1 -> 开启积分/1
  Error/1 -> Zero-Order Hold/1, Derivative/1
  Memory/1 -> 输出达到正限幅时积分不再增大/1(Err), 输出达到负限幅时积分不再减小/1(Err), Subsystem/2(Err)
  Memory1/1 -> 输出达到负限幅时积分不再减小/2(Out), 输出达到正限幅时积分不再增大/2(Out)

== system engine/节气门方案/发电机/反馈量滤波 ==
  Signal : Inport
  Constant2 : Constant  Value=Frq
  Gain : Gain  Gain=2*pi
  d_Smp_LPF6 : cstblocks/Linear Parameter Varying/Varying Lowpass Filter  N=Order
      settings: SourceProductName=Control System Toolbox
  Output : Outport
  wires:
  Gain/1 -> d_Smp_LPF6/2
  Signal/1 -> d_Smp_LPF6/1
  Constant2/1 -> Gain/1
  d_Smp_LPF6/1 -> Output/1  "Is"

== system engine/节气门方案/发电机/设定值响应速度 ==
  Signal : Inport
  Constant2 : Constant  Value=Frq
  Gain : Gain  Gain=2*pi
  d_Smp_LPF6 : cstblocks/Linear Parameter Varying/Varying Lowpass Filter  N=Order
      settings: SourceProductName=Control System Toolbox
  Output : Outport
  wires:
  Gain/1 -> d_Smp_LPF6/2
  Signal/1 -> d_Smp_LPF6/1
  Constant2/1 -> Gain/1
  d_Smp_LPF6/1 -> Output/1  "Is"

== system engine/节气门方案/汽油机/EngineBackup ==
  Clock : Clock
  Constant : Constant  Value=100
  Constant1 : Constant
  Constant2 : Constant
  Gain : Gain  Gain=1/10^5  SaturateOnIntegerOverflow=on  OutDataTypeStr=Inherit: Same as input  ParamDataTypeStr=Inherit: Same as input
  Gain1 : Gain  Gain=180  SaturateOnIntegerOverflow=on  OutDataTypeStr=Inherit: Same as input  ParamDataTypeStr=Inherit: Same as input
  Gain2 : Gain  Gain=1/14.7  SaturateOnIntegerOverflow=on  OutDataTypeStr=Inherit: Same as input  ParamDataTypeStr=Inherit: Same as input
  Product : Product  Inputs=/*  SaturateOnIntegerOverflow=on  OutDataTypeStr=Inherit: Same as first input
  Rate Limiter : RateLimiter  RisingSlewLimit=0.02  FallingSlewLimit=-0.02  SampleTimeMode=inherited
  Scope{,1..3} (4 alike) : Scope
  Step : Step  Time=5  Before=0.4  After=0.2  SampleTime=0
  Step1 : Step  Time=7  Before=0.2  After=0.4  SampleTime=0
  Switch : Switch  Threshold=20  SaturateOnIntegerOverflow=on
  air model : Subsystem
  crank : Subsystem
  fuel : Subsystem
  wires:
  Rate Limiter/1 -> Gain1/1, fuel/1(a_throttle), air model/2(a_throttle), Scope3/1  "节气门开度"
  Step1/1 -> Switch/3
  Step/1 -> Switch/1
  Constant1/1 -> crank/3(Lambda)
  air model/1("dM_air_engine ") -> Product/2
  air model/2(dMfu) -> Scope2/1, fuel/3(dMfu)
  Product/1 -> Gain2/1
  fuel/1(dMf) -> Product/1, crank/1(dMf)
  Gain1/1 -> crank/5(throttle)
  air model/3(Pm_pa) -> Gain/1
  Constant2/1 -> crank/2(theta)
  Switch/1 -> Rate Limiter/1
  crank/1(n) -> air model/1(n), fuel/2(n), Scope/1
  Constant/1 -> crank/6(load)
  Clock/1 -> Switch/2
  Gain2/1 -> Scope1/1
  Gain/1 -> crank/4(Pm)

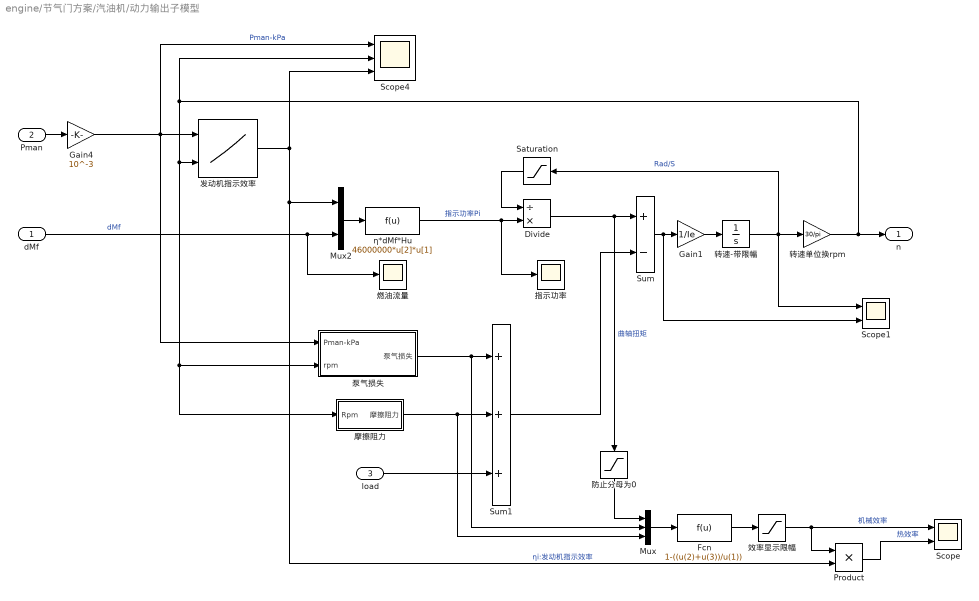
== system engine/节气门方案/汽油机/动力输出子模型 ==
  dMf : Inport
  Pman : Inport  Port=2
  load : Inport  Port=3
  Divide : Product  Inputs=/*
  Fcn : Fcn  Expr=1-((u(2)+u(3))/u(1))
  Gain1 : Gain  Gain=1/Ie  SaturateOnIntegerOverflow=on  OutDataTypeStr=Inherit: Same as input  ParamDataTypeStr=Inherit: Same as input
  Gain4 : Gain  Gain=10^-3  SaturateOnIntegerOverflow=on  OutDataTypeStr=Inherit: Same as input  ParamDataTypeStr=Inherit: Same as input
  Mux : Mux  Inputs=3
  Mux2 : Mux  Inputs=2
  Product : Product
  Saturation : Saturate  UpperLimit=1e8  LowerLimit=0.01
  Scope : Scope  NumInputPorts=2
  Scope1 : Scope  NumInputPorts=2
  Scope4 : Scope  NumInputPorts=3
  Sum : Sum  Inputs=+-  SaturateOnIntegerOverflow=on
  Sum1 : Sum  Inputs=+++  SaturateOnIntegerOverflow=on
  η*dMf*Hu : Fcn  Expr=46000000*u[2]*u[1]
  发动机指示效率 : Lookup_n-D  BreakpointsForDimension1=[0,10,20,50,70,90,110,120]  BreakpointsForDimension2=[-250,0,250,500,750,1000,2000,3000,4000,5000,6000,7000]  Table=reshape([0,0,0,0,0,0,0,0,0,0,0,0,0,0,0,0,0,0.11391,0.27091,0.24318,0.2625,0.25725,0.252,0.2415,0,0.12027,0.31212,0.35455,0.37485,0.3675,0.36435,0.35175,0,0.12452,0.32545,0.39477,0.40425,0.4011,0.3927,0.37485,0,0.12706,0.33068,0.39341,0.4053,0.40425,0.3948,0.378,0,0.133,0.34485,0.39614,0.40635,0.4053,0.39795,0.3843,0,0.13568,0.35939,0.39477,0.40635,0.40635,0.399,0.3864,0,0.13023,0.37432,0.40425,0.4053,0.40425,0.399,0.38745,0,0.12068,0.38,0.4032,0.40425,0.3969,0.3927,0.38535,0,0.11433,0.37295,0.39375,0.40005,0.3927,0.38745,0.37695,0,0.10364,0.35576,0.3759,0.38115,0.3801,0.3759,0.3696],8,12)  DiagnosticForOutOfRangeInput=Warning  InternalRulePriority=Speed  RndMeth=Simplest  InputSameDT=on
  指示功率 : Scope
  摩擦阻力 : Subsystem
  效率显示限幅 : Saturate  UpperLimit=1  LowerLimit=0
  泵气损失 : Subsystem
  燃油流量 : Scope
  转速-带限幅 : Integrator  InitialCondition=104  LimitOutput=on  UpperSaturationLimit=628  LowerSaturationLimit=-10
  转速单位换rpm : Gain  Gain=30/pi  SaturateOnIntegerOverflow=on  OutDataTypeStr=Inherit: Same as input  ParamDataTypeStr=Inherit: Same as input
  防止分母为0 : Saturate  UpperLimit=inf  LowerLimit=1e-6
  n : Outport
  wires:
  效率显示限幅/1 -> Scope/1, Product/1  "机械效率"
  防止分母为0/1 -> Mux/1
  Saturation/1 -> Divide/1
  Product/1 -> Scope/2  "热效率"
  Fcn/1 -> 效率显示限幅/1
  Mux/1 -> Fcn/1
  Divide/1 -> Sum/1, 防止分母为0/1  "曲轴扭矩"
  泵气损失/1(泵气损失) -> Sum1/1, Mux/2
  Pman/1 -> Gain4/1
  Gain4/1 -> Scope4/1, 发动机指示效率/1, 泵气损失/1(Pman-kPa)  "Pman-kPa"
  摩擦阻力/1(摩擦阻力) -> Sum1/2, Mux/3
  dMf/1 -> 燃油流量/1, Mux2/2  "dMf"
  发动机指示效率/1 -> Mux2/1, Product/2, Scope4/3  "ηi:发动机指示效率"
  Mux2/1 -> η*dMf*Hu/1
  η*dMf*Hu/1 -> Divide/2, 指示功率/1  "指示功率Pi"
  Sum/1 -> Gain1/1, Scope1/2
  Gain1/1 -> 转速-带限幅/1
  转速单位换rpm/1 -> Scope4/2, 发动机指示效率/2, 泵气损失/2(rpm), 摩擦阻力/1(Rpm), n/1
  load/1 -> Sum1/3
  Sum1/1 -> Sum/2
  转速-带限幅/1 -> Saturation/1, 转速单位换rpm/1, Scope1/1  "Rad/S"

== system engine/节气门方案/汽油机/喷油控制、燃油模型 ==
  note: X: 喷射的燃油中沉积于壁面的比例
      | tau: 油膜蒸发时间常数
  note: dMfu: 通过当前发动机进气量和理论空燃比计算的理论喷油量
  note: 根据dMfu、tau和X
      | 计算所需燃油喷射流量dMfi
  note: dMf: 进入气缸的燃油流量
  note: X: 喷射的燃油中沉积于壁面的比例
  note: dMfi: 燃油喷射流量
  note: tau: 油膜蒸发时间常数
  a_throttle : Inport
  n : Inport  Port=2
  dMfu : Inport  Port=3
  Scope::tau:X : Scope  NumInputPorts=2
  喷油控制算法 : Subsystem
  查表得当前X和tau : Subsystem
  燃油模型 : Subsystem
  dMf : Outport
  wires:
  喷油控制算法/1(dMfi) -> 燃油模型/3(dMfi)
  dMfu/1 -> 喷油控制算法/3(dMfu)
  查表得当前X和tau/1(X) -> 燃油模型/1(X), Scope::tau:X/2, 喷油控制算法/1(X)
  a_throttle/1 -> 查表得当前X和tau/1(throttle)
  n/1 -> 查表得当前X和tau/2(n)
  燃油模型/1(dMf) -> dMf/1
  查表得当前X和tau/2(tau) -> 燃油模型/2(tau), Scope::tau:X/1, 喷油控制算法/2(tau)

== system engine/节气门方案/汽油机/输入滤波 ==
  Signal : Inport
  Constant2 : Constant  Value=Frq
  Gain : Gain  Gain=2*pi
  d_Smp_LPF6 : cstblocks/Linear Parameter Varying/Varying Lowpass Filter  N=Order
      settings: SourceProductName=Control System Toolbox
  Output : Outport
  wires:
  Gain/1 -> d_Smp_LPF6/2
  Signal/1 -> d_Smp_LPF6/1
  Constant2/1 -> Gain/1
  d_Smp_LPF6/1 -> Output/1  "Is"

== system engine/节气门方案/汽油机/进气模型 ==
  note: Mat: 进入进气歧管的空气质量流动速率
      | Map: 离开进气管进入燃烧室的空气质量流动速率
      | Pman: 进气歧管绝对压力(kPa)
  note: Map = n*Vd*η-vol*Pman/(120*R*Tman)
  n : Inport
  a_throttle : Inport  Port=2
  理论空燃比 : Gain  Gain=1/14.7  SaturateOnIntegerOverflow=on  OutDataTypeStr=Inherit: Same as input  ParamDataTypeStr=Inherit: Same as input
  节气门体子模型 : Subsystem
  进气歧管子模型 : Subsystem
  进气门口模型 : Subsystem
  "dM_air_engine " : Outport
  dMfu : Outport  Port=2
  Pman : Outport  Port=3
  wires:
  n/1 -> 进气门口模型/2(n)
  进气门口模型/1(Map) -> "dM_air_engine "/1, 理论空燃比/1, 进气歧管子模型/2(dM_air_engine)  "Map"
  理论空燃比/1 -> dMfu/1
  a_throttle/1 -> 节气门体子模型/1(a_throttle)
  进气歧管子模型/1(Pman) -> Pman/1, 节气门体子模型/2(Pman), 进气门口模型/1(Pman)
  节气门体子模型/1(dM_throttle) -> 进气歧管子模型/1(dM_throttle)  "Mat"

== system engine/节气门方案/电动油门/滞后 ==
  Signal : Inport
  Constant2 : Constant  Value=Frq
  Gain : Gain  Gain=2*pi
  d_Smp_LPF6 : cstblocks/Linear Parameter Varying/Varying Lowpass Filter  N=Order
      settings: SourceProductName=Control System Toolbox
  Output : Outport
  wires:
  Gain/1 -> d_Smp_LPF6/2
  Signal/1 -> d_Smp_LPF6/1
  Constant2/1 -> Gain/1
  d_Smp_LPF6/1 -> Output/1  "Is"

== system engine/节气门方案/转速-功率标定/Subsystem1 ==
  发电功率 : Inport
  Derivative : Derivative  CoefficientInTFapproximation=0.1
  LPF : Subsystem  mask{Frq=1, Order=5}
      mask prompts: Frq "Frq_Set"; Order "Order_Set"
  Saturation : Saturate  UpperLimit=1500  LowerLimit=0
  控制斜率 : Outport
  wires:
  LPF/1(Output) -> Saturation/1
  Saturation/1 -> 控制斜率/1  "控制斜率"
  Derivative/1 -> LPF/1(Signal)
  发电功率/1 -> Derivative/1

== system engine/节气门方案/转速闭环/微分 ==
  Err : Inport
  Derivative : Derivative  CoefficientInTFapproximation=0.1
  微分滤波1 : Subsystem  mask{Frq=fc_Set, Order=3}
      mask prompts: Frq "Frq_Set"; Order "Order_Set"
  dErr : Outport
  wires:
  Derivative/1 -> dErr/1
  微分滤波1/1(Output) -> Derivative/1
  Err/1 -> 微分滤波1/1(Signal)

== system engine/节气门方案/转速闭环/积分控制 ==
  note: 转速快速增大时积分不增大
      | 转速快速减小时积分不减小
  Error : Inport
  Output : Inport  Port=2
  Derivative : Derivative  CoefficientInTFapproximation=0.1
  Memory : Memory
  Memory1 : Memory
  Product1 : Product  Inputs=3
  Scope : Scope  NumInputPorts=3
  Subsystem : Subsystem
  Zero-Order Hold : ZeroOrderHold  SampleTime=0.01
  Zero-Order Hold1 : ZeroOrderHold  SampleTime=0.01
  Zero-Order Hold2 : ZeroOrderHold  SampleTime=0.01
  输出达到正限幅时积分不再增大 : Subsystem
  输出达到负限幅时积分不再减小 : Subsystem
  开启积分 : Outport
  wires:
  Subsystem/1(启动积分) -> Product1/1, Scope/1  "斜率限制"
  Zero-Order Hold1/1 -> Subsystem/1(dErr)
  Zero-Order Hold2/1 -> Memory1/1
  Derivative/1 -> Zero-Order Hold1/1
  Zero-Order Hold/1 -> Memory/1
  输出达到正限幅时积分不再增大/1(启动积分) -> Product1/2, Scope/2  "正限幅限制"
  输出达到负限幅时积分不再减小/1(启动积分) -> Product1/3, Scope/3  "负限幅限制"
  Output/1 -> Zero-Order Hold2/1
  Product1/1 -> 开启积分/1
  Error/1 -> Zero-Order Hold/1, Derivative/1
  Memory/1 -> 输出达到正限幅时积分不再增大/1(Err), 输出达到负限幅时积分不再减小/1(Err), Subsystem/2(Err)
  Memory1/1 -> 输出达到负限幅时积分不再减小/2(Out), 输出达到正限幅时积分不再增大/2(Out)

== system engine/转速方案/功率反馈补偿/功率反馈滤波 ==
  Signal : Inport
  Constant2 : Constant  Value=Frq
  Gain : Gain  Gain=2*pi
  d_Smp_LPF6 : cstblocks/Linear Parameter Varying/Varying Lowpass Filter  N=Order
      settings: SourceProductName=Control System Toolbox
  Output : Outport
  wires:
  d_Smp_LPF6/1 -> Output/1  "Is"
  Constant2/1 -> Gain/1
  Signal/1 -> d_Smp_LPF6/1
  Gain/1 -> d_Smp_LPF6/2

== system engine/转速方案/功率反馈补偿/功率反馈补偿后滤波 ==
  Signal : Inport
  Constant2 : Constant  Value=Frq
  Gain : Gain  Gain=2*pi
  d_Smp_LPF6 : cstblocks/Linear Parameter Varying/Varying Lowpass Filter  N=Order
      settings: SourceProductName=Control System Toolbox
  Output : Outport
  wires:
  Gain/1 -> d_Smp_LPF6/2
  Signal/1 -> d_Smp_LPF6/1
  Constant2/1 -> Gain/1
  d_Smp_LPF6/1 -> Output/1  "Is"

== system engine/转速方案/功率闭环/微分 ==
  Err : Inport
  Derivative : Derivative  CoefficientInTFapproximation=0.1
  微分滤波1 : Subsystem  mask{Frq=fc_Set, Order=1}
      mask prompts: Frq "Frq_Set"; Order "Order_Set"
  dErr : Outport
  wires:
  Derivative/1 -> dErr/1
  微分滤波1/1(Output) -> Derivative/1
  Err/1 -> 微分滤波1/1(Signal)

== system engine/转速方案/功率闭环/积分控制 ==
  note: 功率快速增大时积分不增大
      | 功率快速减小时积分不减小
  Error : Inport
  Output : Inport  Port=2
  Derivative : Derivative  CoefficientInTFapproximation=0.1
  Memory : Memory
  Memory1 : Memory
  Product1 : Product  Inputs=3
  Scope : Scope  NumInputPorts=3
  Subsystem : Subsystem
  Zero-Order Hold : ZeroOrderHold  SampleTime=0.01
  Zero-Order Hold1 : ZeroOrderHold  SampleTime=0.01
  Zero-Order Hold2 : ZeroOrderHold  SampleTime=0.01
  输出达到正限幅时积分不再增大 : Subsystem
  输出达到负限幅时积分不再减小 : Subsystem
  开启积分 : Outport
  wires:
  Subsystem/1(启动积分) -> Product1/1, Scope/1  "斜率限制"
  Zero-Order Hold1/1 -> Subsystem/1(dErr)
  Zero-Order Hold2/1 -> Memory1/1
  Derivative/1 -> Zero-Order Hold1/1
  Zero-Order Hold/1 -> Memory/1
  输出达到正限幅时积分不再增大/1(启动积分) -> Product1/2, Scope/2  "正限幅限制"
  输出达到负限幅时积分不再减小/1(启动积分) -> Product1/3, Scope/3  "负限幅限制"
  Output/1 -> Zero-Order Hold2/1
  Product1/1 -> 开启积分/1
  Error/1 -> Zero-Order Hold/1, Derivative/1
  Memory/1 -> 输出达到正限幅时积分不再增大/1(Err), 输出达到负限幅时积分不再减小/1(Err), Subsystem/2(Err)
  Memory1/1 -> 输出达到负限幅时积分不再减小/2(Out), 输出达到正限幅时积分不再增大/2(Out)

== system engine/转速方案/发电机/设定值响应速度 ==
  Signal : Inport
  Constant2 : Constant  Value=Frq
  Gain : Gain  Gain=2*pi
  d_Smp_LPF6 : cstblocks/Linear Parameter Varying/Varying Lowpass Filter  N=Order
      settings: SourceProductName=Control System Toolbox
  Output : Outport
  wires:
  d_Smp_LPF6/1 -> Output/1  "Is"
  Constant2/1 -> Gain/1
  Signal/1 -> d_Smp_LPF6/1
  Gain/1 -> d_Smp_LPF6/2

== system engine/转速方案/汽油机/EngineBackup ==
  Clock : Clock
  Constant : Constant  Value=100
  Constant1 : Constant
  Constant2 : Constant
  Gain : Gain  Gain=1/10^5  SaturateOnIntegerOverflow=on  OutDataTypeStr=Inherit: Same as input  ParamDataTypeStr=Inherit: Same as input
  Gain1 : Gain  Gain=180  SaturateOnIntegerOverflow=on  OutDataTypeStr=Inherit: Same as input  ParamDataTypeStr=Inherit: Same as input
  Gain2 : Gain  Gain=1/14.7  SaturateOnIntegerOverflow=on  OutDataTypeStr=Inherit: Same as input  ParamDataTypeStr=Inherit: Same as input
  Product : Product  Inputs=/*  SaturateOnIntegerOverflow=on  OutDataTypeStr=Inherit: Same as first input
  Rate Limiter : RateLimiter  RisingSlewLimit=0.02  FallingSlewLimit=-0.02  SampleTimeMode=inherited
  Scope{,1..3} (4 alike) : Scope
  Step : Step  Time=5  Before=0.4  After=0.2  SampleTime=0
  Step1 : Step  Time=7  Before=0.2  After=0.4  SampleTime=0
  Switch : Switch  Threshold=20  SaturateOnIntegerOverflow=on
  air model : Subsystem
  crank : Subsystem
  fuel : Subsystem
  wires:
  Gain/1 -> crank/4(Pm)
  Gain2/1 -> Scope1/1
  Clock/1 -> Switch/2
  Constant/1 -> crank/6(load)
  crank/1(n) -> Scope/1, fuel/2(n), air model/1(n)
  Switch/1 -> Rate Limiter/1
  Constant2/1 -> crank/2(theta)
  air model/3(Pm_pa) -> Gain/1
  Gain1/1 -> crank/5(throttle)
  fuel/1(dMf) -> crank/1(dMf), Product/1
  Product/1 -> Gain2/1
  air model/2(dMfu) -> fuel/3(dMfu), Scope2/1
  air model/1("dM_air_engine ") -> Product/2
  Constant1/1 -> crank/3(Lambda)
  Step/1 -> Switch/1
  Step1/1 -> Switch/3
  Rate Limiter/1 -> Scope3/1, air model/2(a_throttle), fuel/1(a_throttle), Gain1/1  "节气门开度"

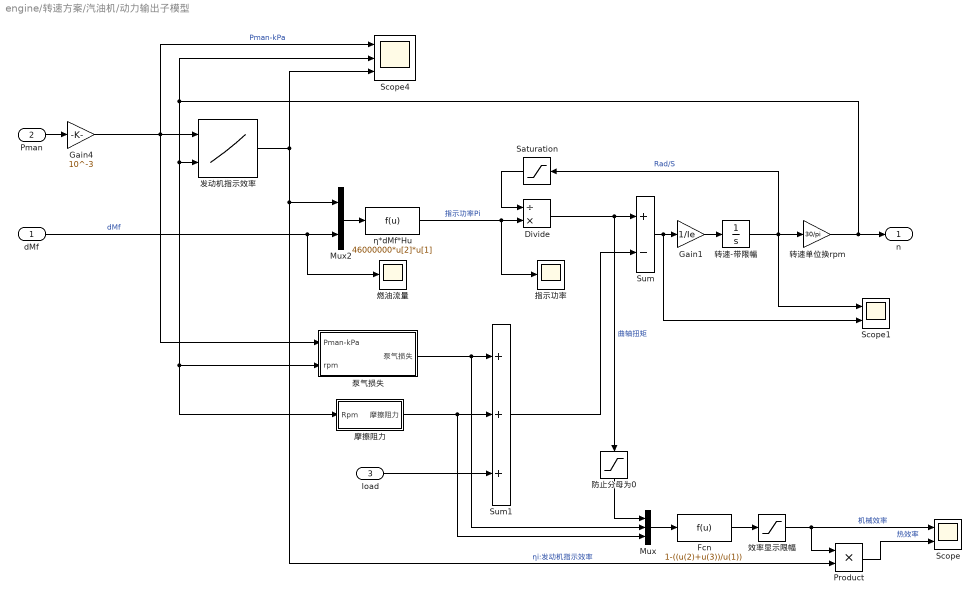
== system engine/转速方案/汽油机/动力输出子模型 ==
  dMf : Inport
  Pman : Inport  Port=2
  load : Inport  Port=3
  Divide : Product  Inputs=/*
  Fcn : Fcn  Expr=1-((u(2)+u(3))/u(1))
  Gain1 : Gain  Gain=1/Ie  SaturateOnIntegerOverflow=on  OutDataTypeStr=Inherit: Same as input  ParamDataTypeStr=Inherit: Same as input
  Gain4 : Gain  Gain=10^-3  SaturateOnIntegerOverflow=on  OutDataTypeStr=Inherit: Same as input  ParamDataTypeStr=Inherit: Same as input
  Mux : Mux  Inputs=3
  Mux2 : Mux  Inputs=2
  Product : Product
  Saturation : Saturate  UpperLimit=1e8  LowerLimit=0.01
  Scope : Scope  NumInputPorts=2
  Scope1 : Scope  NumInputPorts=2
  Scope4 : Scope  NumInputPorts=3
  Sum : Sum  Inputs=+-  SaturateOnIntegerOverflow=on
  Sum1 : Sum  Inputs=+++  SaturateOnIntegerOverflow=on
  η*dMf*Hu : Fcn  Expr=46000000*u[2]*u[1]
  发动机指示效率 : Lookup_n-D  BreakpointsForDimension1=[0,10,20,50,70,90,110,120]  BreakpointsForDimension2=[-250,0,250,500,750,1000,2000,3000,4000,5000,6000,7000]  Table=reshape([0,0,0,0,0,0,0,0,0,0,0,0,0,0,0,0,0,0.11391,0.27091,0.24318,0.2625,0.25725,0.252,0.2415,0,0.12027,0.31212,0.35455,0.37485,0.3675,0.36435,0.35175,0,0.12452,0.32545,0.39477,0.40425,0.4011,0.3927,0.37485,0,0.12706,0.33068,0.39341,0.4053,0.40425,0.3948,0.378,0,0.133,0.34485,0.39614,0.40635,0.4053,0.39795,0.3843,0,0.13568,0.35939,0.39477,0.40635,0.40635,0.399,0.3864,0,0.13023,0.37432,0.40425,0.4053,0.40425,0.399,0.38745,0,0.12068,0.38,0.4032,0.40425,0.3969,0.3927,0.38535,0,0.11433,0.37295,0.39375,0.40005,0.3927,0.38745,0.37695,0,0.10364,0.35576,0.3759,0.38115,0.3801,0.3759,0.3696],8,12)  DiagnosticForOutOfRangeInput=Warning  InternalRulePriority=Speed  RndMeth=Simplest  InputSameDT=on
  指示功率 : Scope
  摩擦阻力 : Subsystem
  效率显示限幅 : Saturate  UpperLimit=1  LowerLimit=0
  泵气损失 : Subsystem
  燃油流量 : Scope
  转速-带限幅 : Integrator  InitialCondition=104  LimitOutput=on  UpperSaturationLimit=628  LowerSaturationLimit=-10
  转速单位换rpm : Gain  Gain=30/pi  SaturateOnIntegerOverflow=on  OutDataTypeStr=Inherit: Same as input  ParamDataTypeStr=Inherit: Same as input
  防止分母为0 : Saturate  UpperLimit=inf  LowerLimit=1e-6
  n : Outport
  wires:
  转速-带限幅/1 -> Scope1/1, 转速单位换rpm/1, Saturation/1  "Rad/S"
  Sum1/1 -> Sum/2
  load/1 -> Sum1/3
  转速单位换rpm/1 -> n/1, 摩擦阻力/1(Rpm), 泵气损失/2(rpm), 发动机指示效率/2, Scope4/2
  Gain1/1 -> 转速-带限幅/1
  Sum/1 -> Scope1/2, Gain1/1
  η*dMf*Hu/1 -> 指示功率/1, Divide/2  "指示功率Pi"
  Mux2/1 -> η*dMf*Hu/1
  发动机指示效率/1 -> Scope4/3, Product/2, Mux2/1  "ηi:发动机指示效率"
  dMf/1 -> Mux2/2, 燃油流量/1  "dMf"
  摩擦阻力/1(摩擦阻力) -> Mux/3, Sum1/2
  Gain4/1 -> 泵气损失/1(Pman-kPa), 发动机指示效率/1, Scope4/1  "Pman-kPa"
  Pman/1 -> Gain4/1
  泵气损失/1(泵气损失) -> Mux/2, Sum1/1
  Divide/1 -> 防止分母为0/1, Sum/1  "曲轴扭矩"
  Mux/1 -> Fcn/1
  Fcn/1 -> 效率显示限幅/1
  Product/1 -> Scope/2  "热效率"
  Saturation/1 -> Divide/1
  防止分母为0/1 -> Mux/1
  效率显示限幅/1 -> Product/1, Scope/1  "机械效率"

== system engine/转速方案/汽油机/喷油控制、燃油模型 ==
  note: tau: 油膜蒸发时间常数
  note: dMfi: 燃油喷射流量
  note: X: 喷射的燃油中沉积于壁面的比例
  note: dMf: 进入气缸的燃油流量
  note: 根据dMfu、tau和X
      | 计算所需燃油喷射流量dMfi
  note: dMfu: 通过当前发动机进气量和理论空燃比计算的理论喷油量
  note: X: 喷射的燃油中沉积于壁面的比例
      | tau: 油膜蒸发时间常数
  a_throttle : Inport
  n : Inport  Port=2
  dMfu : Inport  Port=3
  Scope::tau:X : Scope  NumInputPorts=2
  喷油控制算法 : Subsystem
  查表得当前X和tau : Subsystem
  燃油模型 : Subsystem
  dMf : Outport
  wires:
  查表得当前X和tau/2(tau) -> 喷油控制算法/2(tau), Scope::tau:X/1, 燃油模型/2(tau)
  燃油模型/1(dMf) -> dMf/1
  n/1 -> 查表得当前X和tau/2(n)
  a_throttle/1 -> 查表得当前X和tau/1(throttle)
  查表得当前X和tau/1(X) -> 喷油控制算法/1(X), Scope::tau:X/2, 燃油模型/1(X)
  dMfu/1 -> 喷油控制算法/3(dMfu)
  喷油控制算法/1(dMfi) -> 燃油模型/3(dMfi)

== system engine/转速方案/汽油机/输入滤波 ==
  Signal : Inport
  Constant2 : Constant  Value=Frq
  Gain : Gain  Gain=2*pi
  d_Smp_LPF6 : cstblocks/Linear Parameter Varying/Varying Lowpass Filter  N=Order
      settings: SourceProductName=Control System Toolbox
  Output : Outport
  wires:
  d_Smp_LPF6/1 -> Output/1  "Is"
  Constant2/1 -> Gain/1
  Signal/1 -> d_Smp_LPF6/1
  Gain/1 -> d_Smp_LPF6/2

== system engine/转速方案/汽油机/进气模型 ==
  note: Map = n*Vd*η-vol*Pman/(120*R*Tman)
  note: Mat: 进入进气歧管的空气质量流动速率
      | Map: 离开进气管进入燃烧室的空气质量流动速率
      | Pman: 进气歧管绝对压力(kPa)
  n : Inport
  a_throttle : Inport  Port=2
  理论空燃比 : Gain  Gain=1/14.7  SaturateOnIntegerOverflow=on  OutDataTypeStr=Inherit: Same as input  ParamDataTypeStr=Inherit: Same as input
  节气门体子模型 : Subsystem
  进气歧管子模型 : Subsystem
  进气门口模型 : Subsystem
  "dM_air_engine " : Outport
  dMfu : Outport  Port=2
  Pman : Outport  Port=3
  wires:
  节气门体子模型/1(dM_throttle) -> 进气歧管子模型/1(dM_throttle)  "Mat"
  进气歧管子模型/1(Pman) -> 进气门口模型/1(Pman), 节气门体子模型/2(Pman), Pman/1
  a_throttle/1 -> 节气门体子模型/1(a_throttle)
  理论空燃比/1 -> dMfu/1
  进气门口模型/1(Map) -> 进气歧管子模型/2(dM_air_engine), 理论空燃比/1, "dM_air_engine "/1  "Map"
  n/1 -> 进气门口模型/2(n)

== system engine/转速方案/油门信号控制/功率反馈滤波 ==
  Signal : Inport
  Constant2 : Constant  Value=Frq
  Gain : Gain  Gain=2*pi
  d_Smp_LPF6 : cstblocks/Linear Parameter Varying/Varying Lowpass Filter  N=Order
      settings: SourceProductName=Control System Toolbox
  Output : Outport
  wires:
  Gain/1 -> d_Smp_LPF6/2
  Signal/1 -> d_Smp_LPF6/1
  Constant2/1 -> Gain/1
  d_Smp_LPF6/1 -> Output/1  "Is"

== system engine/转速方案/油门信号控制/转速稳定检查 ==
  转速反馈 : Inport
  Abs : Abs
  Constant : Constant  Value=-10
  Constant1 : Constant
  Constant2 : Constant  Value=0
  Constant3 : Constant
  Derivative : Derivative
  Integrator : Integrator  LimitOutput=on  UpperSaturationLimit=1.1  LowerSaturationLimit=0
  Switch : Switch  Criteria=u2 > Threshold  Threshold=200
  Switch1 : Switch  Criteria=u2 > Threshold  Threshold=1
  Zero-Order Hold : ZeroOrderHold  SampleTime=0.01
  Zero-Order Hold1 : ZeroOrderHold  SampleTime=0.01
  转速反馈滤波 : Subsystem  mask{Frq=5, Order=5}
      mask prompts: Frq "Frq_Set"; Order "Order_Set"
  转速稳定标志 : Outport
  wires:
  Integrator/1 -> Zero-Order Hold1/1
  Constant1/1 -> Switch/3
  Constant2/1 -> Switch1/1
  转速反馈滤波/1(Output) -> Derivative/1
  Derivative/1 -> Zero-Order Hold/1  "转速变化率"
  Switch/1 -> Integrator/1
  Zero-Order Hold1/1 -> Switch1/2
  Zero-Order Hold/1 -> Abs/1
  Switch1/1 -> 转速稳定标志/1  "转速稳定标志"
  Constant/1 -> Switch/1
  Abs/1 -> Switch/2
  Constant3/1 -> Switch1/3
  转速反馈/1 -> 转速反馈滤波/1(Signal)

== system engine/转速方案/转速闭环/微分 ==
  Err : Inport
  Derivative : Derivative  CoefficientInTFapproximation=0.1
  微分滤波1 : Subsystem  mask{Frq=fc_Set, Order=1}
      mask prompts: Frq "Frq_Set"; Order "Order_Set"
  dErr : Outport
  wires:
  Err/1 -> 微分滤波1/1(Signal)
  微分滤波1/1(Output) -> Derivative/1
  Derivative/1 -> dErr/1

== system engine/转速方案/转速闭环/积分控制 ==
  note: 转速快速增大时积分不增大
      | 转速快速减小时积分不减小
  Error : Inport
  Output : Inport  Port=2
  Derivative : Derivative  CoefficientInTFapproximation=0.1
  Memory : Memory
  Memory1 : Memory
  Product1 : Product  Inputs=3
  Scope : Scope  NumInputPorts=3
  Subsystem : Subsystem
  Zero-Order Hold : ZeroOrderHold  SampleTime=0.01
  Zero-Order Hold1 : ZeroOrderHold  SampleTime=0.01
  Zero-Order Hold2 : ZeroOrderHold  SampleTime=0.01
  输出达到正限幅时积分不再增大 : Subsystem
  输出达到负限幅时积分不再减小 : Subsystem
  开启积分 : Outport
  wires:
  Memory1/1 -> 输出达到正限幅时积分不再增大/2(Out), 输出达到负限幅时积分不再减小/2(Out)
  Memory/1 -> Subsystem/2(Err), 输出达到负限幅时积分不再减小/1(Err), 输出达到正限幅时积分不再增大/1(Err)
  Error/1 -> Derivative/1, Zero-Order Hold/1
  Product1/1 -> 开启积分/1
  Output/1 -> Zero-Order Hold2/1
  输出达到负限幅时积分不再减小/1(启动积分) -> Scope/3, Product1/3  "负限幅限制"
  输出达到正限幅时积分不再增大/1(启动积分) -> Scope/2, Product1/2  "正限幅限制"
  Zero-Order Hold/1 -> Memory/1
  Derivative/1 -> Zero-Order Hold1/1
  Zero-Order Hold2/1 -> Memory1/1
  Zero-Order Hold1/1 -> Subsystem/1(dErr)
  Subsystem/1(启动积分) -> Scope/1, Product1/1  "斜率限制"

== system engine/节气门方案/功率闭环/微分/微分滤波1 ==
  Signal : Inport
  Constant2 : Constant  Value=Frq
  Gain : Gain  Gain=2*pi
  d_Smp_LPF6 : cstblocks/Linear Parameter Varying/Varying Lowpass Filter  N=Order
      settings: SourceProductName=Control System Toolbox
  Output : Outport
  wires:
  d_Smp_LPF6/1 -> Output/1  "Is"
  Constant2/1 -> Gain/1
  Signal/1 -> d_Smp_LPF6/1
  Gain/1 -> d_Smp_LPF6/2

== system engine/节气门方案/功率闭环/积分控制/Subsystem ==
  dErr : Inport
  Err : Inport  Port=2
  Abs : Abs
  Constant10 : Constant
  Constant3 : Constant  Value=0
  Constant4 : Constant
  Memory2 : Memory
  Product : Product
  Switch1 : Switch  Criteria=u2 > Threshold  Threshold=dPWR
  Switch6 : Switch  Criteria=u2 > Threshold
  启动积分 : Outport
  wires:
  Switch1/1 -> 启动积分/1
  Err/1 -> Product/2
  Switch6/1 -> Switch1/1
  Product/1 -> Memory2/1
  Constant3/1 -> Switch6/3
  Abs/1 -> Switch1/2
  Constant4/1 -> Switch1/3
  Constant10/1 -> Switch6/1
  dErr/1 -> Abs/1, Product/1
  Memory2/1 -> Switch6/2

== system engine/节气门方案/功率闭环/积分控制/输出达到正限幅时积分不再增大 ==
  Err : Inport
  Out : Inport  Port=2
  Constant : Constant  Value=Acc_p
  Constant2 : Constant
  Constant5 : Constant  Value=0
  Constant6 : Constant
  Sum2 : Sum  Inputs=-+|
  Switch2 : Switch  Criteria=u2 > Threshold
  Switch3 : Switch  Criteria=u2 > Threshold
  启动积分 : Outport
  wires:
  Err/1 -> Switch2/2
  Switch3/1 -> Switch2/1
  Constant/1 -> Sum2/1
  Constant2/1 -> Switch2/3
  Constant6/1 -> Switch3/3
  Out/1 -> Sum2/2
  Sum2/1 -> Switch3/2
  Switch2/1 -> 启动积分/1
  Constant5/1 -> Switch3/1

== system engine/节气门方案/功率闭环/积分控制/输出达到负限幅时积分不再减小 ==
  Err : Inport
  Out : Inport  Port=2
  Constant1 : Constant
  Constant7 : Constant  Value=0
  Constant8 : Constant
  Constant9 : Constant  Value=-Acc_n
  Sum3 : Sum  Inputs=+-|
  Switch4 : Switch  Criteria=u2 > Threshold
  Switch5 : Switch  Criteria=u2 > Threshold
  启动积分 : Outport
  wires:
  Constant8/1 -> Switch5/3
  Switch4/1 -> 启动积分/1
  Constant7/1 -> Switch5/1
  Constant9/1 -> Sum3/1
  Constant1/1 -> Switch4/1
  Err/1 -> Switch4/2
  Out/1 -> Sum3/2
  Switch5/1 -> Switch4/3
  Sum3/1 -> Switch5/2

== system engine/节气门方案/汽油机/EngineBackup/air model ==
  n : Inport
  a_throttle : Inport  Port=2
  Gain : Gain  Gain=1/14.7  SaturateOnIntegerOverflow=on  OutDataTypeStr=Inherit: Same as input  ParamDataTypeStr=Inherit: Same as input
  Subsystem : Subsystem
  Subsystem1 : Subsystem
  Subsystem2 : Subsystem
  "dM_air_engine " : Outport
  dMfu : Outport  Port=2
  Pm_pa : Outport  Port=3
  wires:
  Subsystem1/1(dM_throttle) -> Subsystem2/1(dM_throttle)
  Subsystem2/1(Pm_pa) -> Subsystem/1(Pm), Subsystem1/2(Pm_pa), Pm_pa/1
  a_throttle/1 -> Subsystem1/1(a_throttle)
  Gain/1 -> dMfu/1
  Subsystem/1(dM_air_engine) -> Subsystem2/2(dM_air_engine), Gain/1, "dM_air_engine "/1
  n/1 -> Subsystem/2(n)
